simulink model "LinModelMracScaled"  (R2023b)
settings: Solver=ode23s  StartTime=0.0  StopTime=10  RelTol=1e-3
values from neighbouring files (symbols this model uses):
  A_mat = [0,     1,                  0 ... (first row only)    [mracShell.m]    (also in mracShellScaled.m)
  Am = [0,        1,          0 ... (first row only)    [mracShell.m]    (also in mracShellScaled.m)
  B_mat = [0; 0; (-4*beta_e/Ve)*(Kq*Kv)]    [mracShell.m]    (also in mracShellScaled.m)
  Bm = [0; 0; bm3]    [mracShell.m]    (also in mracShellScaled.m)
  gamma_L = gamma_M    (= 1e-12)    [mracShell.m]    (also in mracShellScaled.m = gamma_M)
  gamma_M = 1e-12    [mracShell.m]    (also in mracShellScaled.m = 1 / (norm(B_z)^2 * norm(P_z)))
  PB_vec_z = P_z * B_z    [mracShellScaled.m]
  T_inv = diag([1/x1_scale, 1/x2_scale, 1/x3_scale])    [mracShellScaled.m]
settings Model: Creator=snr  LastModifiedBy=snr

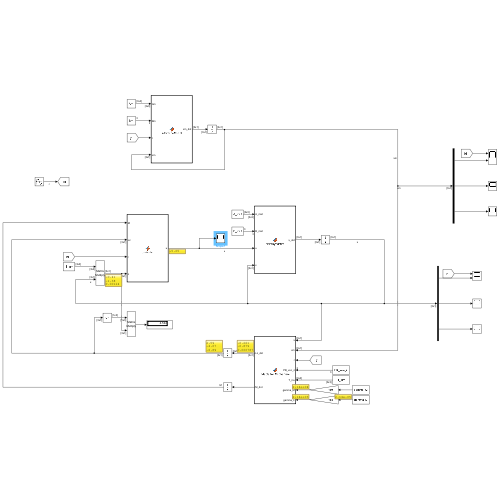
[thumbnail: Simulink's stored preview of the top-level diagram]
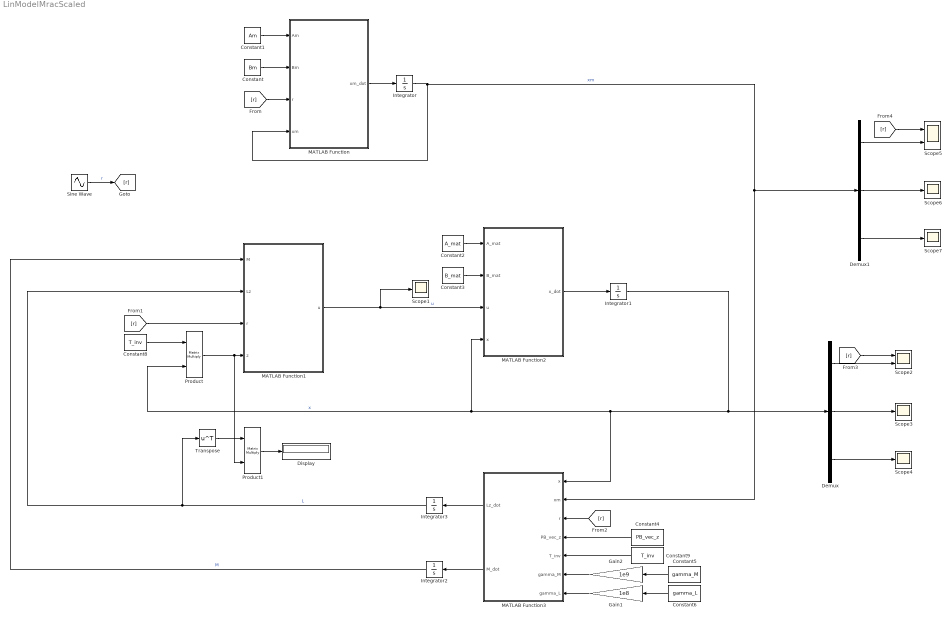
== system LinModelMracScaled ==
  Constant : Constant  Value=Bm
  Constant1 : Constant  Value=Am
  Constant2 : Constant  Value=A_mat
  Constant3 : Constant  Value=B_mat
  Constant4 : Constant  Value=PB_vec_z
  Constant5 : Constant  Value=gamma_M
  Constant6 : Constant  Value=gamma_L
  Constant8 : Constant  Value=T_inv
  Constant9 : Constant  Value=T_inv
  Demux : Demux  Outputs=3
  Demux1 : Demux  Outputs=3
  Display : Display
  Gain1 : Gain  Gain=1e8
  Gain2 : Gain  Gain=1e9
  Integrator : Integrator  InitialCondition=[0;0;0]
  Integrator1 : Integrator  InitialCondition=[0;0;0]
  Integrator2 : Integrator
  Integrator3 : Integrator
  MATLAB Function : MATLAB Function  TreatAsAtomicUnit=on
  MATLAB Function1 : MATLAB Function  TreatAsAtomicUnit=on
  MATLAB Function2 : MATLAB Function  TreatAsAtomicUnit=on
  MATLAB Function3 : MATLAB Function  TreatAsAtomicUnit=on
  Product : Product  Multiplication=Matrix(*)
  Product1 : Product  Multiplication=Matrix(*)
  Scope{1,3..4,6..7} (5 alike) : Scope
  Scope2 : Scope  NumInputPorts=2
  Scope5 : Scope  NumInputPorts=2
  Sine Wave : Sin  Amplitude=80e-3  SampleTime=0
  Transpose : Math  Operator=transpose
  wires:
  MATLAB Function/1(xm_dot) -> Integrator/1
  Sine Wave/1 -> [r]  "r"
  [r] -> MATLAB Function/3(r)
  Constant/1 -> MATLAB Function/2(Bm)
  Constant1/1 -> MATLAB Function/1(Am)
  [r] -> MATLAB Function1/3(r)
  MATLAB Function2/1(x_dot) -> Integrator1/1
  Integrator1/1 -> MATLAB Function2/4(x), Product/2, MATLAB Function3/1(x), Demux/1  "x"
  Constant2/1 -> MATLAB Function2/1(A_mat)
  Constant3/1 -> MATLAB Function2/2(B_mat)
  Constant4/1 -> MATLAB Function3/4(PB_vec_z)
  Constant6/1 -> Gain1/1
  MATLAB Function3/2(M_dot) -> Integrator2/1
  MATLAB Function3/1(Lz_dot) -> Integrator3/1
  Integrator3/1 -> Transpose/1, MATLAB Function1/2(Lz)  "L"
  Integrator2/1 -> MATLAB Function1/1(M)  "M"
  [r] -> MATLAB Function3/3(r)
  Demux/1 -> Scope2/2
  Demux/2 -> Scope3/1
  Demux/3 -> Scope4/1
  Constant8/1 -> Product/1
  Product/1 -> Product1/2, MATLAB Function1/4(z)
  MATLAB Function1/1(u) -> Scope1/1, MATLAB Function2/3(u)  "u"
  Constant9/1 -> MATLAB Function3/5(T_inv)
  Gain1/1 -> MATLAB Function3/7(gamma_L)
  [r] -> Scope2/1
  Demux1/1 -> Scope5/2
  Demux1/3 -> Scope7/1
  [r] -> Scope5/1
  Integrator/1 -> MATLAB Function3/2(xm), Demux1/1, MATLAB Function/4(xm)  "xm"
  Demux1/2 -> Scope6/1
  Gain2/1 -> MATLAB Function3/6(gamma_M)
  Constant5/1 -> Gain2/1
  Transpose/1 -> Product1/1
  Product1/1 -> Display/1

== matlab function LinModelMracScaled/MATLAB Function1 ==
  data: M input; u output; Lz input; r input; z input
function u = controller(M, Lz, r, z)
    % Kontrol kanunu (fiziksel koordinatlara geri dön)
    % u = M*r - Lz'*z = M*r - Lz'*(T_inv*x)
    u   = M * r - Lz' * z;
end

% Note
% L -> (1,n)
% x -> (n,1)

% M -> (1,1)
% r -> (1,1)

== matlab function LinModelMracScaled/MATLAB Function ==
  data: Am input; xm_dot output; Bm input; r input; xm input
function xm_dot = referenceModel(Am, Bm, r, xm)

xm_dot = Am*xm + Bm*r;

== matlab function LinModelMracScaled/MATLAB Function2 ==
  data: A_mat input; B_mat input; u input; x_dot output size=[3,1]; x input
function x_dot = plantDynamics(A_mat, B_mat, u, x)
    x_dot = A_mat*x + B_mat*u; %[3,3] x [3,1] + [3,1]x[1,1]
end

== matlab function LinModelMracScaled/MATLAB Function3 ==
  data: x input; xm input; r input; Lz_dot output; PB_vec_z input; T_inv input; gamma_M input; gamma_L input; M_dot output
function [Lz_dot, M_dot] = adaptationMechanism(x, xm, r, PB_vec_z, T_inv, gamma_M, gamma_L)
% Simülasyon içinde (her ODE adımında):
z   = T_inv * x;          % fiziksel → ölçeklendirilmiş
zm  = T_inv * xm;

e_z = zm - z;             % ölçeklendirilmiş hata

chi = PB_vec_z' * e_z;   % skaler

% Adaptasyon (ölçeklendirilmiş L ile çalış)
M_dot  = +gamma_M * chi * r;
Lz_dot = -gamma_L * chi * z;   % L_z ölçeklendirilmiş    

end

% Note
% L -> (1,n)
% x -> (n,1)

% M -> (1,1)
% r -> (1,1)
